simulink model "filtro_LP_temperatura"  (R2021a)
settings: Solver=VariableStepAuto  StartTime=0.0  StopTime=10.0  RelTol=1e-3
undefined symbols (not defined in the file): taub_Ts
settings Model: Creator=fhlla  LastModifiedBy=fhlla

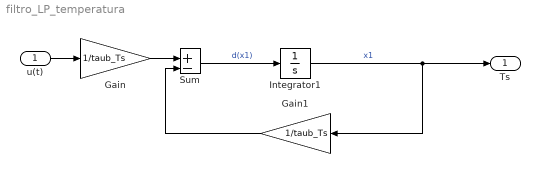
== system filtro_LP_temperatura ==
  u(t) : Inport
  Gain : Gain  Gain=1/taub_Ts
  Gain1 : Gain  Gain=1/taub_Ts
  Integrator1 : Integrator  InitialCondition=40
  Sum : Sum  Inputs=|+|-
  Ts : Outport
  wires:
  Gain1/1 -> Sum/2
  Integrator1/1 -> Ts/1, Gain1/1  "x1"
  u(t)/1 -> Gain/1
  Gain/1 -> Sum/1
  Sum/1 -> Integrator1/1  "d(x1)"
